simulink model "Nine_level_MCI_PMSM_Control"  (R2025a)
settings: Solver=VariableStepAuto  StartTime=0.0  StopTime=1  RelTol=1e-3
undefined symbols (not defined in the file or in its folder): Ion, Lithium
libraries: spsIGBTDiodeLib x48, spsCurrentMeasurementLib x18, spsBreakerLib x12, spsBatteryLib x12, spsVoltageMeasurementLib x6, spsRMSLib x3, slpidlib x1, spsGroundLib x1, spsPermanentMagnetSynchronousMachineLib x1, simulink x1, spsThreePhaseVIMeasurementLib x1, spspowerguiLib x1
(part 2 of 2)

== system Nine_level_MCI_PMSM_Control/9 LEVEL H BRIDGE INVERTER2/MODULE 4 ==
  note: MODULE 1
  g1 : Inport
  g2 : Inport  Port=2
  g3 : Inport  Port=3
  g4 : Inport  Port=4
  IGBT/Diode{,1..3} (4 alike) : spsIGBTDiodeLib/IGBT//Diode  Ron=1e-3  Rs=1e5  Cs=inf  Measurements=on
  Mux : Mux
  + : PMIOPort  Side=Left
  - : PMIOPort  Port=2  Side=Left
  output + : PMIOPort  Port=3  Side=Right
  output - : PMIOPort  Port=4  Side=Right
  switches : Outport
  wires:
  g1/1 -> IGBT/Diode/1
  IGBT/Diode2/1 -> Mux/2
  IGBT/Diode3/1 -> Mux/4
  IGBT/Diode/1 -> Mux/1
  IGBT/Diode1/1 -> Mux/3
  Mux/1 -> switches/1
  g2/1 -> IGBT/Diode3/1
  g3/1 -> IGBT/Diode2/1
  g4/1 -> IGBT/Diode1/1
  connections:
  IGBT/Diode/RConn1 -- output +/RConn1 -- IGBT/Diode2/LConn1
  IGBT/Diode1/RConn1 -- output -/RConn1 -- IGBT/Diode3/LConn1
  IGBT/Diode3/RConn1 -- IGBT/Diode2/RConn1 -- -/RConn1
  IGBT/Diode/LConn1 -- IGBT/Diode1/LConn1 -- +/RConn1

== matlab function Nine_level_MCI_PMSM_Control/Controller/MATLAB Function3 ==
  data: L input; G1 output; G2 output; G3 output; G4 output; G5 output; G6 output; G7 output; G8 output; G9 output; G10 output; G11 output; G12 output; G13 output; G14 output; G15 output; G16 output
function [G1,G2,G3,G4,G5,G6,G7,G8,G9,G10,G11,G12,G13,G14,G15,G16] = CHB9_Gating(L)
%#codegen
% Input: L ∈ {-4,-3,-2,-1,0,1,2,3,4}
% Output: 16 gate signals for 4 H-bridges (4 per bridge)

% Initialize all gate pulses to 0
G1=0; G2=0; G3=0; G4=0;
G5=0; G6=0; G7=0; G8=0;
G9=0; G10=0; G11=0; G12=0;
G13=0; G14=0; G15=0; G16=0;

switch L
    case 4  % +4Vdc = + + + +
        [G1,G2,G3,G4]     = deal(1,1,0,0);
        [G5,G6,G7,G8]     = deal(1,1,0,0);
        [G9,G10,G11,G12]  = deal(1,1,0,0);
        [G13,G14,G15,G16] = deal(1,1,0,0);

    case 3  % +3Vdc = + + + 0
        [G1,G2,G3,G4]     = deal(1,1,0,0);
        [G5,G6,G7,G8]     = deal(1,1,0,0);
        [G9,G10,G11,G12]  = deal(1,1,0,0);
        [G13,G14,G15,G16] = deal(0,1,1,0);

    case 2  % +2Vdc = + + 0 0
        [G1,G2,G3,G4]     = deal(1,1,0,0);
        [G5,G6,G7,G8]     = deal(1,1,0,0);
        [G9,G10,G11,G12]  = deal(0,1,1,0);
        [G13,G14,G15,G16] = deal(0,1,1,0);

    case 1  % +1Vdc = + 0 0 0
        [G1,G2,G3,G4]     = deal(1,1,0,0);
        [G5,G6,G7,G8]     = deal(0,1,1,0);
        [G9,G10,G11,G12]  = deal(0,1,1,0);
        [G13,G14,G15,G16] = deal(0,1,1,0);

    case 0  % 0 = 0 + 0 + 0 + 0
        [G1,G2,G3,G4]     = deal(0,1,1,0);
        [G5,G6,G7,G8]     = deal(0,1,1,0);
        [G9,G10,G11,G12]  = deal(0,1,1,0);
        [G13,G14,G15,G16] = deal(0,1,1,0);

    case -1 % -1Vdc = - + 0 0 0
        [G1,G2,G3,G4]     = deal(0,0,1,1);
        [G5,G6,G7,G8]     = deal(0,1,1,0);
        [G9,G10,G11,G12]  = deal(0,1,1,0);
        [G13,G14,G15,G16] = deal(0,1,1,0);

    case -2 % -2Vdc = - - 0 0
        [G1,G2,G3,G4]     = deal(0,0,1,1);
        [G5,G6,G7,G8]     = deal(0,0,1,1);
        [G9,G10,G11,G12]  = deal(0,1,1,0);
        [G13,G14,G15,G16] = deal(0,1,1,0);

    case -3 % -3Vdc = - - - 0
        [G1,G2,G3,G4]     = deal(0,0,1,1);
        [G5,G6,G7,G8]     = deal(0,0,1,1);
        [G9,G10,G11,G12]  = deal(0,0,1,1);
        [G13,G14,G15,G16] = deal(0,1,1,0);

    case -4 % -4Vdc = - - - -
        [G1,G2,G3,G4]     = deal(0,0,1,1);
        [G5,G6,G7,G8]     = deal(0,0,1,1);
        [G9,G10,G11,G12]  = deal(0,0,1,1);
        [G13,G14,G15,G16] = deal(0,0,1,1);
end
end

== matlab function Nine_level_MCI_PMSM_Control/Controller/Habc to refernce current ==
  data: Ha input; sign_a output; Hb input; Hc input; sign_b output; sign_c output; I_ref input
function [sign_a,sign_b,sign_c] = fcn(Ha,Hb,Hc,I_ref)

if (Ha==1 && Hb==0 && Hc==1)
    sign_a=I_ref;
    sign_b=0;
    sign_c=-I_ref;

elseif (Ha==1 && Hb==0 && Hc==0)
    sign_a=0;
    sign_b=I_ref;
    sign_c=-I_ref;

elseif (Ha==1 && Hb==1 && Hc==0)
    sign_a=-I_ref;
    sign_b=I_ref;
    sign_c=0;

elseif (Ha==0 && Hb==1 && Hc==0)
    sign_a=-I_ref;
    sign_b=0;
    sign_c=I_ref;

elseif (Ha==0 && Hb==1 && Hc==1)
    sign_a=0;
    sign_b=-I_ref;
    sign_c=I_ref;

elseif (Ha==0 && Hb==0 && Hc==1)
    sign_a=I_ref;
    sign_b=-I_ref;
    sign_c=0;

else 
    sign_a=0;
    sign_b=0;
    sign_c=0;

end

== matlab function Nine_level_MCI_PMSM_Control/Controller/MATLAB Function ==
  data: Ia_err input; La output; Ib_err input; Ic_err input; Lb output; Lc output
function [La, Lb, Lc] = MLH7_Controller(Ia_err, Ib_err, Ic_err)
% Multilevel hysteresis controller for 7-level inverter
% Inputs: phase current errors (A)
% Outputs: quantized level commands (-3..+3)
% Author: Rajagopal & ChatGPT (MCI Project)

% --- Tunable hysteresis thresholds (adjust as needed) ---
Delta1 = 1*0.02;   % inner band (A)
Delta2 = 1*0.05;   % mid band (A)
Delta3 = 1*0.07;
Delta4 = 1*0.09;   % outer band (A)

% Compute level for each phase
La = getLevel(Ia_err, Delta1, Delta2, Delta3,Delta4);
Lb = getLevel(Ib_err, Delta1, Delta2, Delta3,Delta4);
Lc = getLevel(Ic_err, Delta1, Delta2, Delta3,Delta4);

end

function L = getLevel(err, D1, D2, D3, D4)
% Converts current error to level command

if err > D4
    L = -4;
elseif err > D3
    L = -3;
elseif err > D2
    L = -2;
elseif err > D1
    L = -1;
elseif err >= -D1 && err <= D1
    L = 0;
elseif err >= -D2
    L = 1;
elseif err >= -D3
    L = 2;
elseif err >=-D4
    L = 3;
else
    L=4;
end

end

== matlab function Nine_level_MCI_PMSM_Control/Controller/Hall sensor output based on Rotor Angle ==
  data: theta input; Ha output; Hb output; Hc output
function [Ha,Hb,Hc] = fcn(theta)

if (theta>330 && theta<=360) || (theta>=0 && theta<=30)
    Ha=1;
    Hb=0;
    Hc=1;

elseif (theta>30 && theta<=90)
    Ha=1;
    Hb=0;
    Hc=0;
elseif (theta>90 && theta<=150)
    Ha=1;
    Hb=1;
    Hc=0;
elseif (theta>150 && theta<=210)
    Ha=0;
    Hb=1;
    Hc=0;
elseif (theta>210 && theta<=270)
    Ha=0;
    Hb=1;
    Hc=1;
elseif (theta>270 && theta<=330)
    Ha=0;
    Hb=0;
    Hc=1;
else
    Ha=0;
    Hb=0;
    Hc=0;
end

== matlab function Nine_level_MCI_PMSM_Control/Controller/MATLAB Function1 ==
  data: L input; G1 output; G2 output; G3 output; G4 output; G5 output; G6 output; G7 output; G8 output; G9 output; G10 output; G11 output; G12 output; G13 output; G14 output; G15 output; G16 output
function [G1,G2,G3,G4,G5,G6,G7,G8,G9,G10,G11,G12,G13,G14,G15,G16] = CHB9_Gating(L)
%#codegen
% Input: L ∈ {-4,-3,-2,-1,0,1,2,3,4}
% Output: 16 gate signals for 4 H-bridges (4 per bridge)

% Initialize all gate pulses to 0
G1=0; G2=0; G3=0; G4=0;
G5=0; G6=0; G7=0; G8=0;
G9=0; G10=0; G11=0; G12=0;
G13=0; G14=0; G15=0; G16=0;

switch L
    case 4  % +4Vdc = + + + +
        [G1,G2,G3,G4]     = deal(1,1,0,0);
        [G5,G6,G7,G8]     = deal(1,1,0,0);
        [G9,G10,G11,G12]  = deal(1,1,0,0);
        [G13,G14,G15,G16] = deal(1,1,0,0);

    case 3  % +3Vdc = + + + 0
        [G1,G2,G3,G4]     = deal(1,1,0,0);
        [G5,G6,G7,G8]     = deal(1,1,0,0);
        [G9,G10,G11,G12]  = deal(1,1,0,0);
        [G13,G14,G15,G16] = deal(0,1,1,0);

    case 2  % +2Vdc = + + 0 0
        [G1,G2,G3,G4]     = deal(1,1,0,0);
        [G5,G6,G7,G8]     = deal(1,1,0,0);
        [G9,G10,G11,G12]  = deal(0,1,1,0);
        [G13,G14,G15,G16] = deal(0,1,1,0);

    case 1  % +1Vdc = + 0 0 0
        [G1,G2,G3,G4]     = deal(1,1,0,0);
        [G5,G6,G7,G8]     = deal(0,1,1,0);
        [G9,G10,G11,G12]  = deal(0,1,1,0);
        [G13,G14,G15,G16] = deal(0,1,1,0);

    case 0  % 0 = 0 + 0 + 0 + 0
        [G1,G2,G3,G4]     = deal(0,1,1,0);
        [G5,G6,G7,G8]     = deal(0,1,1,0);
        [G9,G10,G11,G12]  = deal(0,1,1,0);
        [G13,G14,G15,G16] = deal(0,1,1,0);

    case -1 % -1Vdc = - + 0 0 0
        [G1,G2,G3,G4]     = deal(0,0,1,1);
        [G5,G6,G7,G8]     = deal(0,1,1,0);
        [G9,G10,G11,G12]  = deal(0,1,1,0);
        [G13,G14,G15,G16] = deal(0,1,1,0);

    case -2 % -2Vdc = - - 0 0
        [G1,G2,G3,G4]     = deal(0,0,1,1);
        [G5,G6,G7,G8]     = deal(0,0,1,1);
        [G9,G10,G11,G12]  = deal(0,1,1,0);
        [G13,G14,G15,G16] = deal(0,1,1,0);

    case -3 % -3Vdc = - - - 0
        [G1,G2,G3,G4]     = deal(0,0,1,1);
        [G5,G6,G7,G8]     = deal(0,0,1,1);
        [G9,G10,G11,G12]  = deal(0,0,1,1);
        [G13,G14,G15,G16] = deal(0,1,1,0);

    case -4 % -4Vdc = - - - -
        [G1,G2,G3,G4]     = deal(0,0,1,1);
        [G5,G6,G7,G8]     = deal(0,0,1,1);
        [G9,G10,G11,G12]  = deal(0,0,1,1);
        [G13,G14,G15,G16] = deal(0,0,1,1);
end
end

== matlab function Nine_level_MCI_PMSM_Control/Controller/MATLAB Function2 ==
  data: L input; G1 output; G2 output; G3 output; G4 output; G5 output; G6 output; G7 output; G8 output; G9 output; G10 output; G11 output; G12 output; G13 output; G14 output; G15 output; G16 output
function [G1,G2,G3,G4,G5,G6,G7,G8,G9,G10,G11,G12,G13,G14,G15,G16] = CHB9_Gating(L)
%#codegen
% Input: L ∈ {-4,-3,-2,-1,0,1,2,3,4}
% Output: 16 gate signals for 4 H-bridges (4 per bridge)

% Initialize all gate pulses to 0
G1=0; G2=0; G3=0; G4=0;
G5=0; G6=0; G7=0; G8=0;
G9=0; G10=0; G11=0; G12=0;
G13=0; G14=0; G15=0; G16=0;

switch L
    case 4  % +4Vdc = + + + +
        [G1,G2,G3,G4]     = deal(1,1,0,0);
        [G5,G6,G7,G8]     = deal(1,1,0,0);
        [G9,G10,G11,G12]  = deal(1,1,0,0);
        [G13,G14,G15,G16] = deal(1,1,0,0);

    case 3  % +3Vdc = + + + 0
        [G1,G2,G3,G4]     = deal(1,1,0,0);
        [G5,G6,G7,G8]     = deal(1,1,0,0);
        [G9,G10,G11,G12]  = deal(1,1,0,0);
        [G13,G14,G15,G16] = deal(0,1,1,0);

    case 2  % +2Vdc = + + 0 0
        [G1,G2,G3,G4]     = deal(1,1,0,0);
        [G5,G6,G7,G8]     = deal(1,1,0,0);
        [G9,G10,G11,G12]  = deal(0,1,1,0);
        [G13,G14,G15,G16] = deal(0,1,1,0);

    case 1  % +1Vdc = + 0 0 0
        [G1,G2,G3,G4]     = deal(1,1,0,0);
        [G5,G6,G7,G8]     = deal(0,1,1,0);
        [G9,G10,G11,G12]  = deal(0,1,1,0);
        [G13,G14,G15,G16] = deal(0,1,1,0);

    case 0  % 0 = 0 + 0 + 0 + 0
        [G1,G2,G3,G4]     = deal(0,1,1,0);
        [G5,G6,G7,G8]     = deal(0,1,1,0);
        [G9,G10,G11,G12]  = deal(0,1,1,0);
        [G13,G14,G15,G16] = deal(0,1,1,0);

    case -1 % -1Vdc = - + 0 0 0
        [G1,G2,G3,G4]     = deal(0,0,1,1);
        [G5,G6,G7,G8]     = deal(0,1,1,0);
        [G9,G10,G11,G12]  = deal(0,1,1,0);
        [G13,G14,G15,G16] = deal(0,1,1,0);

    case -2 % -2Vdc = - - 0 0
        [G1,G2,G3,G4]     = deal(0,0,1,1);
        [G5,G6,G7,G8]     = deal(0,0,1,1);
        [G9,G10,G11,G12]  = deal(0,1,1,0);
        [G13,G14,G15,G16] = deal(0,1,1,0);

    case -3 % -3Vdc = - - - 0
        [G1,G2,G3,G4]     = deal(0,0,1,1);
        [G5,G6,G7,G8]     = deal(0,0,1,1);
        [G9,G10,G11,G12]  = deal(0,0,1,1);
        [G13,G14,G15,G16] = deal(0,1,1,0);

    case -4 % -4Vdc = - - - -
        [G1,G2,G3,G4]     = deal(0,0,1,1);
        [G5,G6,G7,G8]     = deal(0,0,1,1);
        [G9,G10,G11,G12]  = deal(0,0,1,1);
        [G13,G14,G15,G16] = deal(0,0,1,1);
end
end
